simulink library "Vehicle_Axle2_None"  (R2026a)
settings: Solver=VariableStepAuto
libraries: sm_lib x1
Description:
  | Component of Simscape Vehicle Templates Library
  | 
  | Copyright 2018-2026 The MathWorks, Inc.
settings Model: Creator=smiller  LastModifiedBy=smiller

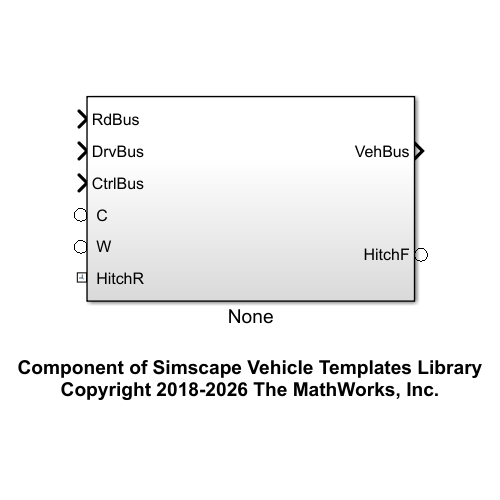
[thumbnail: Simulink's stored preview of the top-level diagram]
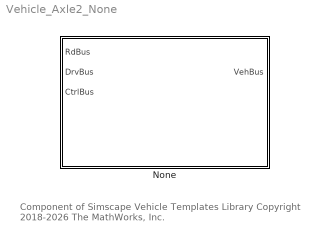
== system Vehicle_Axle2_None ==
  note: Component of Simscape Vehicle Templates Library
      | Copyright 2018-2026 The MathWorks, Inc.
  None : Subsystem  VariantControl=None

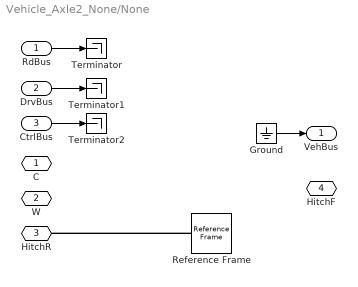
== system Vehicle_Axle2_None/None ==
  "RdBus " : Inport
  "DrvBus " : Inport  Port=2
  "CtrlBus " : Inport  Port=3
  Ground : Ground
  Reference Frame : sm_lib/Frames and Transforms/Reference Frame
  Terminator : Terminator
  Terminator1 : Terminator
  Terminator2 : Terminator
  " C" : PMIOPort  Side=Left
  " W" : PMIOPort  Port=2  Side=Left
  " HitchR" : PMIOPort  Port=3  Side=Left
  HitchF : PMIOPort  Port=4  Side=Right
  " VehBus" : Outport  VectorParamsAs1DForOutWhenUnconnected=off
  wires:
  "RdBus "/1 -> Terminator/1
  "CtrlBus "/1 -> Terminator2/1
  Ground/1 -> " VehBus"/1
  "DrvBus "/1 -> Terminator1/1
  connections:
  Reference Frame/RConn1 -- " HitchR"/RConn1
